simulink model "simulink_4_2"  (R2023b)
settings: Solver=ode5  StartTime=0.0  StopTime=10.0  FixedStep=1/fs  RelTol=1e-3
values from neighbouring files (symbols this model uses):
  fs = 1000    [problem_4_2.m]
settings Model: Creator=sarth  LastModifiedBy=sarth

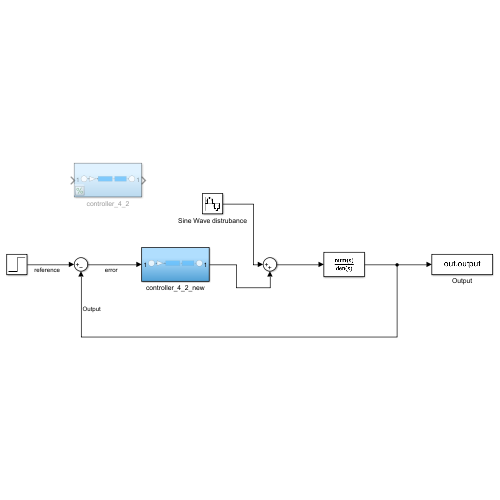
[thumbnail: Simulink's stored preview of the top-level diagram]
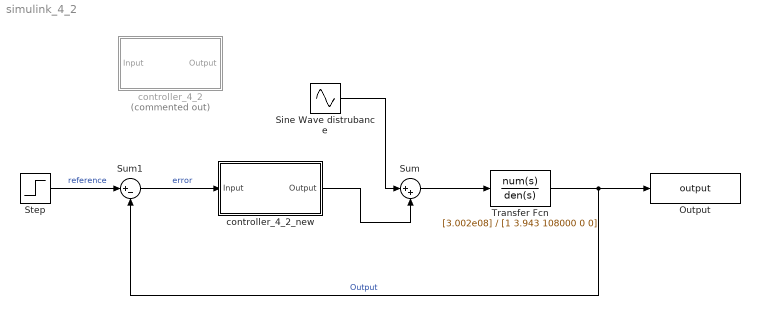
== system simulink_4_2 ==
  Output : ToWorkspace  VariableName=output  SampleTime=-1
  Sine Wave distrubance : Sin  Frequency=12.56  SampleTime=1/fs
  Step : Step  SampleTime=1/fs
  Sum : Sum  Inputs=|++
  Sum1 : Sum  Inputs=|+-
  Transfer Fcn : TransferFcn  Numerator=[3.002e08]  Denominator=[1 3.943 108000 0 0]
  controller_4_2 : Subsystem  Commented=on
  controller_4_2_new : Subsystem
  wires:
  controller_4_2_new/1(Output) -> Sum/2
  Sine Wave distrubance/1 -> Sum/1
  Sum/1 -> Transfer Fcn/1
  Sum1/1 -> controller_4_2_new/1(Input)  "error"
  Step/1 -> Sum1/1  "reference"
  Transfer Fcn/1 -> Output/1, Sum1/2  "Output"

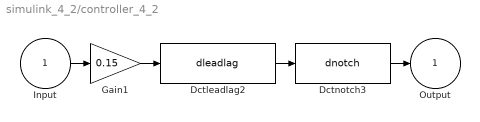
== system simulink_4_2/controller_4_2 ==
  Input : Inport
  Dctleadlag2 : S-Function  FunctionName=dleadlag  Parameters=f_num, f_den, 0.001  SFunctionDeploymentMode=off  EnableBusSupport=off  mask(dctools){f_num=0.9, f_den=16}
      mask prompts: f_num "Zero [Hz]"; f_den "Pole [Hz]"
      mask help: This block implements a discrete time leadlag filter.
      mask Display: disp('DCT leadlag')
  Dctnotch3 : S-Function  FunctionName=dnotch  Parameters=f_num, b_num, f_den, b_den, 0.001  SFunctionDeploymentMode=off  EnableBusSupport=off  mask(dctools){f_num=52.6, b_num=0.1, f_den=52.6, b_den=0.5}
      mask prompts: f_num "Zero [Hz]"; b_num "Damping zero [-]"; f_den "Pole [Hz]"; b_den "Damping pole [-]"
      mask help: This block implements a dicrete time 2nd order notch filter.
      mask Display: disp('DCT notch')
  Gain1 : Gain  Gain=0.15
  Output : Outport
  wires:
  Input/1 -> Gain1/1
  Gain1/1 -> Dctleadlag2/1
  Dctleadlag2/1 -> Dctnotch3/1
  Dctnotch3/1 -> Output/1

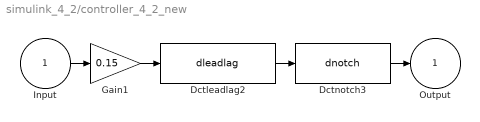
== system simulink_4_2/controller_4_2_new ==
  Input : Inport
  Dctleadlag2 : S-Function  FunctionName=dleadlag  Parameters=f_num, f_den, 0.001  SFunctionDeploymentMode=off  EnableBusSupport=off  mask(dctools){f_num=0.9, f_den=16}
      mask prompts: f_num "Zero [Hz]"; f_den "Pole [Hz]"
      mask help: This block implements a discrete time leadlag filter.
      mask Display: disp('DCT leadlag')
  Dctnotch3 : S-Function  FunctionName=dnotch  Parameters=f_num, b_num, f_den, b_den, 0.001  SFunctionDeploymentMode=off  EnableBusSupport=off  mask(dctools){f_num=52.4, b_num=0.00501, f_den=80, b_den=1}
      mask prompts: f_num "Zero [Hz]"; b_num "Damping zero [-]"; f_den "Pole [Hz]"; b_den "Damping pole [-]"
      mask help: This block implements a dicrete time 2nd order notch filter.
      mask Display: disp('DCT notch')
  Gain1 : Gain  Gain=0.15
  Output : Outport
  wires:
  Input/1 -> Gain1/1
  Gain1/1 -> Dctleadlag2/1
  Dctleadlag2/1 -> Dctnotch3/1
  Dctnotch3/1 -> Output/1
